simulink model "adt_currValGxf"  (R2020a)
settings: Solver=VariableStepAuto  StartTime=0.0  StopTime=10.0  RelTol=1e-3
PreLoadFcn:
  | if exist('tl_preloadfcn','file'), tl_preloadfcn(gcs,'5.1.0.29'); end
PostLoadFcn:
  | if exist('tl_postloadfcn','file'), tl_postloadfcn(gcs,'5.1.0.29'); end
InitFcn:
  | if exist('tlds_init','file'), tlds_init(gcs); end
StartFcn:
  | if exist('tlds_start','file'), tlds_start(gcs); end
StopFcn:
  | if exist('tlds_stop','file'), tlds_stop(gcs); end
libraries: tllib x2
PreSaveFcn:
  | if exist('tl_presavefcn','file'), tl_presavefcn(gcs); end
CloseFcn:
  | if exist('tl_closefcn','file'), tl_closefcn(gcs); end
settings Model: TL_MAIN_DATA={'date', 730486}  TLVersion=5.1.0.29  Creator=developer  LastModifiedBy=developer
settings OptimizationCC: BlockReduction=off  OptimizeBlockIOStorage=off
settings DebuggingCC: BusObjectLabelMismatch=error  StrictBusMsg=ErrorOnBusTreatedAsVector  NonBusSignalsTreatedAsBus=error

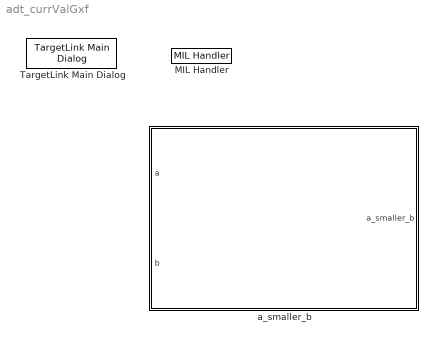
== system adt_currValGxf ==
  MIL Handler : tllib/MIL Handler  data={'date',730486}
      settings: SourceProductName=dSPACE TargetLink common blockset
  TargetLink Main Dialog : tllib/TargetLink Main Dialog  data=[]
      settings: SourceProductName=dSPACE TargetLink common blockset
  a_smaller_b : Subsystem  Tag=TargetLink Simulation Frame  mask(TL_SimFrame){}
      settings: CopyFcn=if exist('tl_copyfcn','file'), tl_copyfcn(gcbh); end  NameChangeFcn=if exist('tl_framenamechangefcn','file'), tl_framenamechangefcn(gcbh); end
      settings: OpenFcn=|
      | if exist('open_tlsubsystem','file')
      |    open_tlsubsystem(gcbh);
      | else
      |    tlsubsystem = ...
      |       find_system(gcb, ...
      |       'LookUnderMasks','on', ...
      |       'FollowLinks','on', ...
      |       'Tag','MIL Subsystem');
      |    open_system(tlsubsystem);
      | end
      mask Display: disp('TargetLink\nModel-\nin-the-loop\nmode')

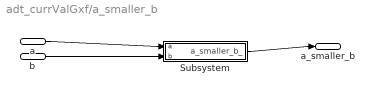
== system adt_currValGxf/a_smaller_b ==
  a : Inport
  b : Inport  Port=2
  Subsystem : Subsystem  mask(TL_Enable){}
      settings: OpenFcn=warndlg(get_param(gcb,'MaskHelp'),'Serious Warning');
      mask Help: This subsystem keeps the TargetLink subsystem (subsystem with TargetLink blocks for production code generation), and is needed for the TargetLink simulation frame to work properly. DO NOT DELETE OR MODIFY IT!
  a_smaller_b : Outport  VectorParamsAs1DForOutWhenUnconnected=off
  wires:
  a/1 -> Subsystem/1(a)
  b/1 -> Subsystem/2(b)
  Subsystem/1(a_smaller_b_) -> a_smaller_b/1

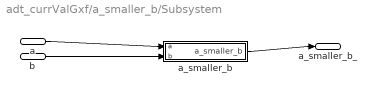
== system adt_currValGxf/a_smaller_b/Subsystem ==
  a : Inport
  b : Inport  Port=2
  a_smaller_b : Subsystem  Tag=MIL Subsystem  mask([]){}
      settings: CopyFcn=if exist('tl_copyfcn','file'), tl_copyfcn(gcbh); end  NameChangeFcn=if exist('tl_namechangefcn','file'), tl_namechangefcn(gcbh); end  DestroyFcn=if exist('update_tl_main_dlg','file'), update_tl_main_dlg('TL_subs_display'); end
      mask Display: disp('TargetLink Subsystem')
  a_smaller_b_ : Outport  VectorParamsAs1DForOutWhenUnconnected=off
  wires:
  a/1 -> a_smaller_b/1(a)
  b/1 -> a_smaller_b/2(b)
  a_smaller_b/1(a_smaller_b) -> a_smaller_b_/1

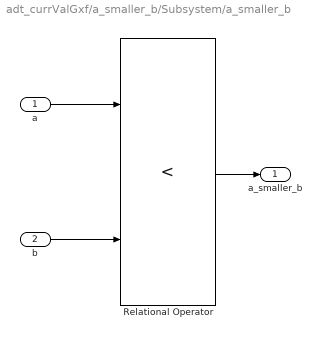
== system adt_currValGxf/a_smaller_b/Subsystem/a_smaller_b ==
  a : Inport  mask(TL_Inport){data={'date',739444.42457197921}}
      settings: DeleteFcn=if exist('delete_tlblock','file')==2,delete_tlblock(gcbh);end  OpenFcn=if exist('tl_open_blockdlg','file')==2,tl_open_blockdlg(gcbh);else,open_system(gcbh,'force');end
      settings: CopyFcn=|
      | if exist('tl_reset_reviewflag','file')==2
      |     tl_reset_reviewflag(gcbh);
      | end
      | if exist('tl_check_ports','file')
      |     tl_check_ports(gcbh);
      | end
      settings: NameChangeFcn=|
      | if exist('rename_tlblock','file')==2,rename_tlblock(gcbh);end
      | if exist('tl_check_ports','file'), tl_check_ports(gcbh); end
      mask Help: eval(['if exist(''tl_online_help'',''file'') == 2, tl_online_help(''Topic'',''TL_Inport''),else, web([''jar:file:///'',matlabroot,''/help/toolbox/simulink/help.jar!/slref/' lower(get_param(gcbh,'Blocktype')) '.html''], ''-helpbrowser''),end'])
      mask Display:
      | [x,y] = tlDrawBrandOnBlockIcon(gcbh);
      | plot(x,y);
  b : Inport  Port=2  mask(TL_Inport){data={'date',739444.42457197921}}
      settings: DeleteFcn=if exist('delete_tlblock','file')==2,delete_tlblock(gcbh);end  OpenFcn=if exist('tl_open_blockdlg','file')==2,tl_open_blockdlg(gcbh);else,open_system(gcbh,'force');end
      settings: CopyFcn=|
      | if exist('tl_reset_reviewflag','file')==2
      |     tl_reset_reviewflag(gcbh);
      | end
      | if exist('tl_check_ports','file')
      |     tl_check_ports(gcbh);
      | end
      settings: NameChangeFcn=|
      | if exist('rename_tlblock','file')==2,rename_tlblock(gcbh);end
      | if exist('tl_check_ports','file'), tl_check_ports(gcbh); end
      mask Help: eval(['if exist(''tl_online_help'',''file'') == 2, tl_online_help(''Topic'',''TL_Inport''),else, web([''jar:file:///'',matlabroot,''/help/toolbox/simulink/help.jar!/slref/' lower(get_param(gcbh,'Blocktype')) '.html''], ''-helpbrowser''),end'])
      mask Display:
      | [x,y] = tlDrawBrandOnBlockIcon(gcbh);
      | plot(x,y);
  Relational Operator : RelationalOperator  Operator=<  OutDataTypeStr=boolean  RndMeth=Simplest  mask(TL_RelationalOperator){data={'date',739444.42620305554}}
      settings: CopyFcn=if exist('copy_tlblock','file')==2,copy_tlblock(gcbh);end  DeleteFcn=if exist('delete_tlblock','file')==2,delete_tlblock(gcbh);end  NameChangeFcn=if exist('rename_tlblock','file')==2,rename_tlblock(gcbh);end  OpenFcn=if exist('tl_open_blockdlg','file')==2,tl_open_blockdlg(gcbh);else,open_system(gcbh,'force');end
      mask Help: eval(['if exist(''tl_online_help'',''file'') == 2, tl_online_help(''Topic'',''TL_RelationalOperator''),else, web([''jar:file:///'',matlabroot,''/help/toolbox/simulink/help.jar!/slref/' lower(get_param(gcbh,'Blocktype')) '.html''], ''-helpbrowser''),end'])
      mask Display:
      | [x,y] = tlDrawBrandOnBlockIcon(gcbh);
      | plot(x,y);
  a_smaller_b : Outport  VectorParamsAs1DForOutWhenUnconnected=off  mask(TL_Outport){data={'output',{'type','Bool'},'date',739444.42703864584}}
      settings: DeleteFcn=if exist('delete_tlblock','file')==2,delete_tlblock(gcbh);end  OpenFcn=if exist('tl_open_blockdlg','file')==2,tl_open_blockdlg(gcbh);else,open_system(gcbh,'force');end
      settings: CopyFcn=|
      | if exist('tl_reset_reviewflag','file')==2
      |     tl_reset_reviewflag(gcbh);
      | end
      | if exist('tl_check_ports','file')
      |     tl_check_ports(gcbh);
      | end
      settings: NameChangeFcn=|
      | if exist('rename_tlblock','file')==2,rename_tlblock(gcbh);end
      | if exist('tl_check_ports','file'), tl_check_ports(gcbh); end
      mask Help: eval(['if exist(''tl_online_help'',''file'') == 2, tl_online_help(''Topic'',''TL_Outport''),else, web([''jar:file:///'',matlabroot,''/help/toolbox/simulink/help.jar!/slref/' lower(get_param(gcbh,'Blocktype')) '.html''], ''-helpbrowser''),end'])
      mask Display:
      | [x,y] = tlDrawBrandOnBlockIcon(gcbh);
      | plot(x,y);
  wires:
  a/1 -> Relational Operator/1
  b/1 -> Relational Operator/2
  Relational Operator/1 -> a_smaller_b/1
